simulink model "light_sensor_calibration_algorithm_test_harness"  (R2013a)
settings: Solver=ode45  StartTime=0.0  StopTime=10.0  RelTol=1e-3
settings Model: Creator=mbiesiad  LastModifiedBy=mbiesiad
settings DataIOCC: SignalLoggingSaveFormat=ModelDataLogs
settings OptimizationCC: ExpressionDepthLimit=2147483647
settings DebuggingCC: MultiTaskDSMMsg=warning  MultiTaskCondExecSysMsg=none  StrictBusMsg=None
settings RTWCC: IncludeERTFirstTime=on

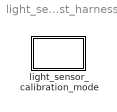
== system light_sensor_calibration_algorithm_test_harness ==
  light_sensor_calibration_mode : Stateflow chart  TreatAsAtomicUnit=on

== stateflow chart light_sensor_calibration_algorithm_test_harness/light_sensor_calibration_mode ==
  state light_sensor_calibration_mode
    during:
